simulink model "sbvf_model_2019b_distributed"  (R2019b)
settings: Solver=VariableStepAuto  StartTime=0.0  StopTime=Tsim  RelTol=1e-3
undefined symbols (not defined in the file): A, A0, Ad, B, C, c, D, F, F_dist, Gdiag, k, K, K0, L_leader, std_dev, x0, x0_leader
libraries: dspindex x102, simulink x1
(part 1 of 2)
settings Model: Creator=andre  LastModifiedBy=frare
settings DebuggingCC: UnconnectedInputMsg=none  UnconnectedOutputMsg=none  UnconnectedLineMsg=none
settings ModelReferenceCC: EnableRefExpFcnMdlSchedulingChecks=off
settings RTWCC: Description=Generic Real-Time Target

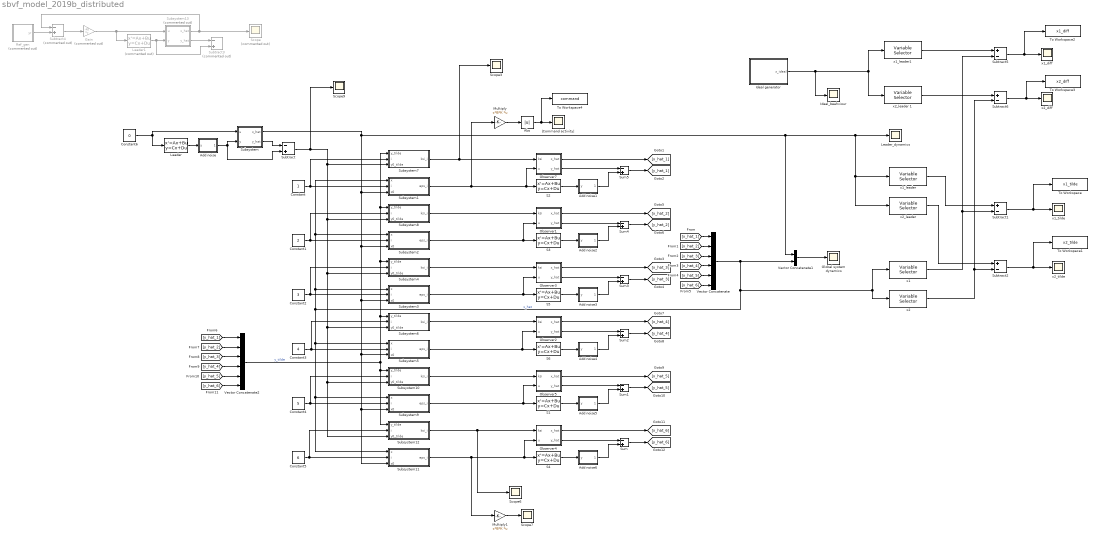
== system sbvf_model_2019b_distributed ==
  Abs : Abs
  Add noise : Subsystem
  "Add noise1 " : Subsystem
  Add noise2 : Subsystem
  Add noise3 : Subsystem
  Add noise4 : Subsystem
  Add noise5 : Subsystem
  Add noise6 : Subsystem
  Constant : Constant
  Constant1 : Constant  Value=2
  Constant2 : Constant  Value=3
  Constant3 : Constant  Value=4
  Constant4 : Constant  Value=5
  Constant5 : Constant  Value=6
  Constant6 : Constant  Value=0
  Gain : Gain  Commented=on  Gain=-K0  Multiplication=Matrix(K*u)
  Global system dynamics : Scope
  "Ideal generator " : Subsystem
  "Ideal_beahviour " : Scope
  Leader : StateSpace  A=A0  B=B  C=C  D=0  InitialCondition=x0_leader
  Leader1 : StateSpace  Commented=on  A=A  B=B  C=C  D=0  InitialCondition=x0_leader
  "Leader_dynamics " : Scope
  Multiply : Gain  Gain=c*B*K  Multiplication=Matrix(K*u)
  Multiply1 : Gain  Gain=c*B*K  Multiplication=Matrix(K*u)
  Observer1 : Subsystem
  Observer2 : Subsystem
  Observer3 : Subsystem
  Observer4 : Subsystem
  Observer5 : Subsystem
  Observer7 : Subsystem
  Ref_gen : Subsystem  Commented=on
  S1 : StateSpace  A=A0  B=c*B*K  C=C  D=D  InitialCondition=x0(:,5)
  S2 : StateSpace  A=A0  B=c*B*K  C=C  D=D  InitialCondition=x0(:,1)
  S3 : StateSpace  A=A0  B=c*B*K  C=C  D=D  InitialCondition=x0(:,2)
  S4 : StateSpace  A=A0  B=c*B*K  C=C  D=D  InitialCondition=x0(:,6)
  S5 : StateSpace  A=A0  B=c*B*K  C=C  D=D  InitialCondition=x0(:,3)
  S6 : StateSpace  A=A0  B=c*B*K  C=C  D=D  InitialCondition=x0(:,4)
  Scope : Scope  Commented=on
  Scope{3,6..7,9} (4 alike) : Scope
  Subsystem : Subsystem
  Subsystem1 : Subsystem
  Subsystem10 : Subsystem
  Subsystem11 : Subsystem
  Subsystem12 : Subsystem
  Subsystem13 : Subsystem  Commented=on
  Subsystem2 : Subsystem
  Subsystem3 : Subsystem
  Subsystem4 : Subsystem
  Subsystem5 : Subsystem
  Subsystem6 : Subsystem
  Subsystem7 : Subsystem
  Subsystem8 : Subsystem
  Subsystem9 : Subsystem
  Subtract : Sum  Inputs=-+
  Subtract{1..2,5..6} (4 alike) : Sum  Inputs=+-
  Subtract3 : Sum  Commented=on  Inputs=-+
  Subtract4 : Sum  Commented=on  Inputs=-+
  Sum{,1..5} (6 alike) : Sum  Inputs=-+
  To Workspace : ToWorkspace  VariableName=x1_tilde  SaveFormat=Timeseries  SampleTime=-1
  To Workspace1 : ToWorkspace  VariableName=x2_tilde  SaveFormat=Timeseries  SampleTime=-1
  To Workspace2 : ToWorkspace  VariableName=x1_diff  SaveFormat=Timeseries  SampleTime=-1
  To Workspace3 : ToWorkspace  VariableName=x2_diff  SaveFormat=Timeseries  SampleTime=-1
  To Workspace4 : ToWorkspace  VariableName=command  SaveFormat=Timeseries  SampleTime=-1
  Vector Concatenate : Concatenate  NumInputs=6  Mode=Multidimensional array  ConcatenateDimension=2
  Vector Concatenate1 : Concatenate  Mode=Multidimensional array  ConcatenateDimension=2
  Vector Concatenate2 : Concatenate  NumInputs=6  Mode=Multidimensional array  ConcatenateDimension=2
  x1 : dspindex/Variable Selector  NumInputs=1  rowsOrCols=Rows  IdxMode=Fixed  Elements=1  ZerOneIdxMode=One-based  errmode=Clip Index  FillMode=on  FillValues=0
  "x1_diff " : Scope
  x1_leader : dspindex/Variable Selector  NumInputs=1  rowsOrCols=Rows  IdxMode=Fixed  Elements=1  ZerOneIdxMode=One-based  errmode=Clip Index  FillMode=on  FillValues=0
  x1_leader1 : dspindex/Variable Selector  NumInputs=1  rowsOrCols=Rows  IdxMode=Fixed  Elements=1  ZerOneIdxMode=One-based  errmode=Clip Index  FillMode=on  FillValues=0
  x1_tilde : Scope
  x2 : dspindex/Variable Selector  NumInputs=1  rowsOrCols=Rows  IdxMode=Fixed  Elements=2  ZerOneIdxMode=One-based  errmode=Clip Index  FillMode=on  FillValues=0
  x2_diff : Scope
  "x2_leader " : dspindex/Variable Selector  NumInputs=1  rowsOrCols=Rows  IdxMode=Fixed  Elements=2  ZerOneIdxMode=One-based  errmode=Clip Index  FillMode=on  FillValues=0
  x2_leader 1 : dspindex/Variable Selector  NumInputs=1  rowsOrCols=Rows  IdxMode=Fixed  Elements=2  ZerOneIdxMode=One-based  errmode=Clip Index  FillMode=on  FillValues=0
  "x2_tilde " : Scope
  "|Command activity| " : Scope
  wires:
  Constant/1 -> Subsystem7/2(i), Subsystem1/2(i)
  Constant1/1 -> Subsystem8/2(i), Subsystem2/2(i)
  Vector Concatenate/1 -> Subsystem1/1(x), Subsystem2/1(x), Subsystem3/1(x), Subsystem11/1(x), Subsystem9/1(x), Subsystem5/1(x), x2/1, x1/1, Vector Concatenate1/2  "x_hat"
  Vector Concatenate1/1 -> Global system dynamics/1
  Constant3/1 -> Subsystem6/2(i), Subsystem5/2(i)
  Constant5/1 -> Subsystem12/2(i), Subsystem11/2(i)
  Constant4/1 -> Subsystem10/2(i), Subsystem9/2(i)
  Constant2/1 -> Subsystem4/2(i), Subsystem3/2(i)
  Subsystem2/1(eps_i) -> S3/1, Observer1/2(u)
  Subsystem3/1(eps_i) -> Observer3/2(u), S5/1
  Subsystem5/1(eps_i) -> S6/1, Observer2/2(u)
  Subsystem9/1(eps_i) -> S1/1, Observer5/2(u)
  Subsystem/2(y_hat) -> Subtract/1
  Subsystem7/1(ksi_i) -> Scope3/1, Observer7/1("ksi ")
  Subsystem10/1(ksi_i) -> Observer5/1("ksi ")
  Subsystem6/1(ksi_i) -> Observer2/1("ksi ")
  Subsystem4/1(ksi_i) -> Observer3/1("ksi ")
  Subsystem8/1(ksi_i) -> Observer1/1("ksi ")
  Observer4/2(y_hat) -> Sum/1
  Observer5/2(y_hat) -> Sum1/1
  Observer2/2(y_hat) -> Sum2/1
  Observer3/2(y_hat) -> Sum3/1
  Observer1/2(y_hat) -> Sum4/1
  Observer7/2(y_hat) -> Sum5/1
  Sum5/1 -> [y_hat_1]
  Observer7/1(x_hat) -> [x_hat_1]
  Observer1/1(x_hat) -> [x_hat_2]
  Sum4/1 -> [y_hat_2]
  Observer3/1(x_hat) -> [x_hat_3]
  Sum3/1 -> [y_hat_3]
  Observer2/1(x_hat) -> [x_hat_4]
  Sum2/1 -> [y_hat_4]
  Observer5/1(x_hat) -> [x_hat_5]
  Sum1/1 -> [y_hat_5]
  Observer4/1(x_hat) -> [x_hat_6]
  Sum/1 -> [y_hat_6]
  [x_hat_1] -> Vector Concatenate/1
  [x_hat_2] -> Vector Concatenate/2
  [x_hat_3] -> Vector Concatenate/3
  [x_hat_4] -> Vector Concatenate/4
  [x_hat_5] -> Vector Concatenate/5
  [x_hat_6] -> Vector Concatenate/6
  [y_hat_2] -> Vector Concatenate2/2
  [y_hat_1] -> Vector Concatenate2/1
  [y_hat_5] -> Vector Concatenate2/5
  [y_hat_3] -> Vector Concatenate2/3
  [y_hat_6] -> Vector Concatenate2/6
  [y_hat_4] -> Vector Concatenate2/4
  Vector Concatenate2/1 -> Subsystem7/1("y_tilde "), Subsystem8/1("y_tilde "), Subsystem4/1("y_tilde "), Subsystem6/1("y_tilde "), Subsystem12/1("y_tilde "), Subsystem10/1("y_tilde ")  "y_tilde"
  Subsystem1/1(eps_i) -> Multiply/1, S2/1, Observer7/2(u)
  Subsystem12/1(ksi_i) -> Observer4/1("ksi "), Scope6/1
  Subsystem11/1(eps_i) -> Multiply1/1, Observer4/2(u), S4/1
  Subtract/1 -> Scope9/1, Subsystem12/3("y0_tilde "), Subsystem10/3("y0_tilde "), Subsystem6/3("y0_tilde "), Subsystem4/3("y0_tilde "), Subsystem8/3("y0_tilde "), Subsystem7/3("y0_tilde ")
  Subsystem/1(x_hat) -> Subsystem11/3(x0), Subsystem9/3(x0), Subsystem5/3(x0), Subsystem3/3(x0), Subsystem2/3(x0), Subsystem1/3(x0), Vector Concatenate1/1, "Leader_dynamics "/1, "x2_leader "/1, x1_leader/1
  x1_leader/1 -> Subtract1/1
  x1/1 -> Subtract5/2, Subtract1/2
  "x2_leader "/1 -> Subtract2/1
  x2/1 -> Subtract6/2, Subtract2/2
  Subtract1/1 -> To Workspace/1, x1_tilde/1
  Constant6/1 -> Subsystem/1(u), Leader/1
  Leader1/1 -> Subtract3/2, Subsystem13/2("y ")
  Subtract4/1 -> Gain/1
  Subsystem13/2(y_hat) -> Subtract3/1
  Subsystem13/1(x_hat) -> Subtract4/1, Scope/1
  Ref_gen/1(yr) -> Subtract4/2
  Gain/1 -> Subsystem13/1(u), Leader1/1
  Subtract2/1 -> To Workspace1/1, "x2_tilde "/1
  "Add noise1 "/1(y_noisy) -> Sum5/2
  Add noise2/1(y_noisy) -> Sum4/2
  Add noise3/1(y_noisy) -> Sum3/2
  Add noise4/1(y_noisy) -> Sum2/2
  Add noise5/1(y_noisy) -> Sum1/2
  Add noise6/1(y_noisy) -> Sum/2
  Add noise/1(y_noisy) -> Subtract/2, Subsystem/2("y ")
  Leader/1 -> Add noise/1(y)
  S3/1 -> Add noise2/1(y)
  S2/1 -> "Add noise1 "/1(y)
  S5/1 -> Add noise3/1(y)
  S6/1 -> Add noise4/1(y)
  S1/1 -> Add noise5/1(y)
  S4/1 -> Add noise6/1(y)
  "Ideal generator "/1("x_ideal ") -> "Ideal_beahviour "/1, x2_leader 1/1, x1_leader1/1
  x1_leader1/1 -> Subtract5/1
  x2_leader 1/1 -> Subtract6/1
  Subtract5/1 -> To Workspace2/1, "x1_diff "/1
  Subtract6/1 -> To Workspace3/1, x2_diff/1
  Multiply/1 -> Abs/1
  Multiply1/1 -> Scope7/1
  Abs/1 -> To Workspace4/1, "|Command activity| "/1

== system sbvf_model_2019b_distributed/Add noise ==
  y : Inport
  Random Number : RandomNumber  SampleTime=0.1
  Sum : Sum  Inputs=|++
  "std_dev(k) " : Gain  Gain=std_dev(k)
  y_noisy : Outport
  wires:
  Random Number/1 -> "std_dev(k) "/1
  y/1 -> Sum/1
  "std_dev(k) "/1 -> Sum/2
  Sum/1 -> y_noisy/1

== system sbvf_model_2019b_distributed/Add noise1  ==
  y : Inport
  Random Number : RandomNumber  SampleTime=0.1
  Sum : Sum  Inputs=|++
  "std_dev(k) " : Gain  Gain=std_dev(k)
  y_noisy : Outport
  wires:
  Random Number/1 -> "std_dev(k) "/1
  y/1 -> Sum/1
  "std_dev(k) "/1 -> Sum/2
  Sum/1 -> y_noisy/1

== system sbvf_model_2019b_distributed/Add noise2 ==
  y : Inport
  Random Number : RandomNumber  SampleTime=0.1
  Sum : Sum  Inputs=|++
  "std_dev(k) " : Gain  Gain=std_dev(k)
  y_noisy : Outport
  wires:
  Random Number/1 -> "std_dev(k) "/1
  y/1 -> Sum/1
  "std_dev(k) "/1 -> Sum/2
  Sum/1 -> y_noisy/1

== system sbvf_model_2019b_distributed/Add noise3 ==
  y : Inport
  Random Number : RandomNumber  SampleTime=0.1
  Sum : Sum  Inputs=|++
  "std_dev(k) " : Gain  Gain=std_dev(k)
  y_noisy : Outport
  wires:
  Random Number/1 -> "std_dev(k) "/1
  y/1 -> Sum/1
  "std_dev(k) "/1 -> Sum/2
  Sum/1 -> y_noisy/1

== system sbvf_model_2019b_distributed/Add noise4 ==
  y : Inport
  Random Number : RandomNumber  SampleTime=0.1
  Sum : Sum  Inputs=|++
  "std_dev(k) " : Gain  Gain=std_dev(k)
  y_noisy : Outport
  wires:
  Random Number/1 -> "std_dev(k) "/1
  y/1 -> Sum/1
  "std_dev(k) "/1 -> Sum/2
  Sum/1 -> y_noisy/1

== system sbvf_model_2019b_distributed/Add noise5 ==
  y : Inport
  Random Number : RandomNumber  SampleTime=0.1
  Sum : Sum  Inputs=|++
  "std_dev(k) " : Gain  Gain=std_dev(k)
  y_noisy : Outport
  wires:
  Random Number/1 -> "std_dev(k) "/1
  y/1 -> Sum/1
  "std_dev(k) "/1 -> Sum/2
  Sum/1 -> y_noisy/1

== system sbvf_model_2019b_distributed/Add noise6 ==
  y : Inport
  Random Number : RandomNumber  SampleTime=0.1
  Sum : Sum  Inputs=|++
  "std_dev(k) " : Gain  Gain=std_dev(k)
  y_noisy : Outport
  wires:
  Random Number/1 -> "std_dev(k) "/1
  y/1 -> Sum/1
  "std_dev(k) "/1 -> Sum/2
  Sum/1 -> y_noisy/1

== system sbvf_model_2019b_distributed/Ideal generator  ==
  Constant7 : Constant  Value=0
  Leader2 : StateSpace  A=A0  B=B  C=C  D=0  InitialCondition=x0_leader
  Subsystem14 : Subsystem
  "x_ideal " : Outport
  wires:
  Constant7/1 -> Subsystem14/1(u), Leader2/1
  Leader2/1 -> Subsystem14/2("y ")
  Subsystem14/1(x_hat) -> "x_ideal "/1

== system sbvf_model_2019b_distributed/Observer1 ==
  "ksi " : Inport
  u : Inport  Port=2
  Add1 : Sum  Inputs=+++
  Gain : Gain  Gain=-c*F_dist  Multiplication=Matrix(K*u)
  Gain1 : Gain  Gain=c*B*K  Multiplication=Matrix(K*u)
  Gain2 : Gain  Gain=A0  Multiplication=Matrix(K*u)
  Gain3 : Gain  Gain=C  Multiplication=Matrix(K*u)
  Integrator : Integrator  InitialCondition=x0(:,2)
  x_hat : Outport
  y_hat : Outport  Port=2
  wires:
  Gain2/1 -> Add1/3
  Gain/1 -> Add1/2
  Integrator/1 -> x_hat/1, Gain2/1, Gain3/1  "x_hat"
  Add1/1 -> Integrator/1
  u/1 -> Gain1/1
  Gain1/1 -> Add1/1
  "ksi "/1 -> Gain/1
  Gain3/1 -> y_hat/1

== system sbvf_model_2019b_distributed/Observer2 ==
  "ksi " : Inport
  u : Inport  Port=2
  Add1 : Sum  Inputs=+++
  Gain : Gain  Gain=-c*F_dist  Multiplication=Matrix(K*u)
  Gain1 : Gain  Gain=c*B*K  Multiplication=Matrix(K*u)
  Gain2 : Gain  Gain=A0  Multiplication=Matrix(K*u)
  Gain3 : Gain  Gain=C  Multiplication=Matrix(K*u)
  Integrator : Integrator  InitialCondition=x0(:,4)
  x_hat : Outport
  y_hat : Outport  Port=2
  wires:
  Gain2/1 -> Add1/3
  Gain/1 -> Add1/2
  Integrator/1 -> x_hat/1, Gain2/1, Gain3/1  "x_hat"
  Add1/1 -> Integrator/1
  u/1 -> Gain1/1
  Gain1/1 -> Add1/1
  "ksi "/1 -> Gain/1
  Gain3/1 -> y_hat/1

== system sbvf_model_2019b_distributed/Observer3 ==
  "ksi " : Inport
  u : Inport  Port=2
  Add1 : Sum  Inputs=+++
  Gain : Gain  Gain=-c*F_dist  Multiplication=Matrix(K*u)
  Gain1 : Gain  Gain=c*B*K  Multiplication=Matrix(K*u)
  Gain2 : Gain  Gain=A0  Multiplication=Matrix(K*u)
  Gain3 : Gain  Gain=C  Multiplication=Matrix(K*u)
  Integrator : Integrator  InitialCondition=x0(:,3)
  x_hat : Outport
  y_hat : Outport  Port=2
  wires:
  Gain2/1 -> Add1/3
  Gain/1 -> Add1/2
  Integrator/1 -> x_hat/1, Gain2/1, Gain3/1  "x_hat"
  Add1/1 -> Integrator/1
  u/1 -> Gain1/1
  Gain1/1 -> Add1/1
  "ksi "/1 -> Gain/1
  Gain3/1 -> y_hat/1

== system sbvf_model_2019b_distributed/Observer4 ==
  "ksi " : Inport
  u : Inport  Port=2
  Add1 : Sum  Inputs=+++
  Gain : Gain  Gain=-c*F_dist  Multiplication=Matrix(K*u)
  Gain1 : Gain  Gain=c*B*K  Multiplication=Matrix(K*u)
  Gain2 : Gain  Gain=A0  Multiplication=Matrix(K*u)
  Gain3 : Gain  Gain=C  Multiplication=Matrix(K*u)
  Integrator : Integrator  InitialCondition=x0(:,6)
  x_hat : Outport
  y_hat : Outport  Port=2
  wires:
  Gain2/1 -> Add1/3
  Gain/1 -> Add1/2
  Integrator/1 -> x_hat/1, Gain2/1, Gain3/1  "x_hat"
  Add1/1 -> Integrator/1
  u/1 -> Gain1/1
  Gain1/1 -> Add1/1
  "ksi "/1 -> Gain/1
  Gain3/1 -> y_hat/1

== system sbvf_model_2019b_distributed/Observer5 ==
  "ksi " : Inport
  u : Inport  Port=2
  Add1 : Sum  Inputs=+++
  Gain : Gain  Gain=-c*F_dist  Multiplication=Matrix(K*u)
  Gain1 : Gain  Gain=c*B*K  Multiplication=Matrix(K*u)
  Gain2 : Gain  Gain=A0  Multiplication=Matrix(K*u)
  Gain3 : Gain  Gain=C  Multiplication=Matrix(K*u)
  Integrator : Integrator  InitialCondition=x0(:,5)
  x_hat : Outport
  y_hat : Outport  Port=2
  wires:
  Gain2/1 -> Add1/3
  Gain/1 -> Add1/2
  Integrator/1 -> x_hat/1, Gain2/1, Gain3/1  "x_hat"
  Add1/1 -> Integrator/1
  u/1 -> Gain1/1
  Gain1/1 -> Add1/1
  "ksi "/1 -> Gain/1
  Gain3/1 -> y_hat/1

== system sbvf_model_2019b_distributed/Observer7 ==
  "ksi " : Inport
  u : Inport  Port=2
  Add1 : Sum  Inputs=+++
  Gain : Gain  Gain=-c*F_dist  Multiplication=Matrix(K*u)
  Gain1 : Gain  Gain=c*B*K  Multiplication=Matrix(K*u)
  Gain2 : Gain  Gain=A0  Multiplication=Matrix(K*u)
  Gain3 : Gain  Gain=C  Multiplication=Matrix(K*u)
  Integrator : Integrator  InitialCondition=x0(:,1)
  x_hat : Outport
  y_hat : Outport  Port=2
  wires:
  Gain2/1 -> Add1/3
  Gain/1 -> Add1/2
  Integrator/1 -> x_hat/1, Gain2/1, Gain3/1  "x_hat"
  Add1/1 -> Integrator/1
  u/1 -> Gain1/1
  Gain1/1 -> Add1/1
  "ksi "/1 -> Gain/1
  Gain3/1 -> y_hat/1

== system sbvf_model_2019b_distributed/Ref_gen ==
  Derivative : Derivative
  Mux : Mux  Inputs=2
  Ramp : simulink/Sources/Ramp  slope=1  start=0  InitialOutput=0
  yr : Outport
  wires:
  Mux/1 -> yr/1
  Ramp/1 -> Derivative/1, Mux/1
  Derivative/1 -> Mux/2

== system sbvf_model_2019b_distributed/Subsystem ==
  u : Inport
  "y " : Inport  Port=2
  Add1 : Sum  Inputs=+++
  Gain : Gain  Gain=c*L_leader  Multiplication=Matrix(K*u)
  Gain1 : Gain  Gain=B  Multiplication=Matrix(K*u)
  Gain2 : Gain  Gain=A0  Multiplication=Matrix(K*u)
  Gain3 : Gain  Gain=C  Multiplication=Matrix(K*u)
  Integrator : Integrator  InitialCondition=x0_leader
  Subtract : Sum  Inputs=-+
  x_hat : Outport
  y_hat : Outport  Port=2
  wires:
  Gain2/1 -> Add1/3
  Gain/1 -> Add1/2
  Integrator/1 -> x_hat/1, Gain3/1, Gain2/1  "x_hat"
  Add1/1 -> Integrator/1  "x_hat_dot"
  u/1 -> Gain1/1
  Gain1/1 -> Add1/1
  "y "/1 -> Subtract/2
  Subtract/1 -> Gain/1
  Gain3/1 -> y_hat/1, Subtract/1

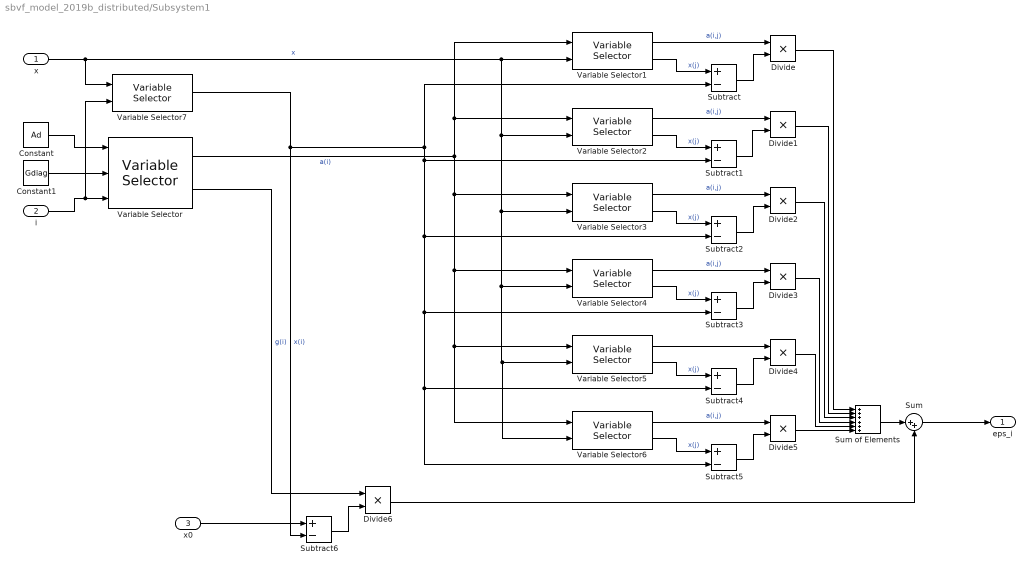
== system sbvf_model_2019b_distributed/Subsystem1 ==
  x : Inport
  i : Inport  Port=2
  x0 : Inport  Port=3
  Constant : Constant  Value=Ad
  Constant1 : Constant  Value=Gdiag
  Divide{,1..6} (7 alike) : Product
  Subtract{,1..6} (7 alike) : Sum  Inputs=+-
  Sum : Sum  Inputs=|++
  Sum of Elements : Sum  Inputs=++++++
  Variable Selector : dspindex/Variable Selector  NumInputs=2  rowsOrCols=Rows  IdxMode=Variable  Elements=[1 3]  ZerOneIdxMode=One-based  errmode=Clip and Warn  FillMode=on  FillValues=0
  Variable Selector1 : dspindex/Variable Selector  NumInputs=2  rowsOrCols=Columns  IdxMode=Fixed  Elements=1  ZerOneIdxMode=One-based  errmode=Generate Error  FillMode=on  FillValues=0
  Variable Selector2 : dspindex/Variable Selector  NumInputs=2  rowsOrCols=Columns  IdxMode=Fixed  Elements=2  ZerOneIdxMode=One-based  errmode=Generate Error  FillMode=on  FillValues=0
  Variable Selector3 : dspindex/Variable Selector  NumInputs=2  rowsOrCols=Columns  IdxMode=Fixed  Elements=3  ZerOneIdxMode=One-based  errmode=Generate Error  FillMode=on  FillValues=0
  Variable Selector4 : dspindex/Variable Selector  NumInputs=2  rowsOrCols=Columns  IdxMode=Fixed  Elements=4  ZerOneIdxMode=One-based  errmode=Generate Error  FillMode=on  FillValues=0
  Variable Selector5 : dspindex/Variable Selector  NumInputs=2  rowsOrCols=Columns  IdxMode=Fixed  Elements=5  ZerOneIdxMode=One-based  errmode=Generate Error  FillMode=on  FillValues=0
  Variable Selector6 : dspindex/Variable Selector  NumInputs=2  rowsOrCols=Columns  IdxMode=Fixed  Elements=6  ZerOneIdxMode=One-based  errmode=Generate Error  FillMode=on  FillValues=0
  Variable Selector7 : dspindex/Variable Selector  NumInputs=1  rowsOrCols=Columns  IdxMode=Variable  Elements=1  ZerOneIdxMode=One-based  errmode=Generate Error  FillMode=on  FillValues=0
  eps_i : Outport
  wires:
  Variable Selector/1 -> Variable Selector3/1, Variable Selector4/1, Variable Selector6/1, Variable Selector5/1, Variable Selector2/1, Variable Selector1/1  "a(i)"
  x/1 -> Variable Selector7/1, Variable Selector2/2, Variable Selector3/2, Variable Selector4/2, Variable Selector6/2, Variable Selector5/2, Variable Selector1/2  "x"
  Constant/1 -> Variable Selector/1
  i/1 -> Variable Selector7/2, Variable Selector/3
  Variable Selector1/1 -> Divide/1  "a(i,j)"
  Variable Selector1/2 -> Subtract/1  "x(j)"
  Subtract/1 -> Divide/2
  Variable Selector2/2 -> Subtract1/1  "x(j)"
  Variable Selector2/1 -> Divide1/1  "a(i,j)"
  Subtract1/1 -> Divide1/2
  Variable Selector3/1 -> Divide2/1  "a(i,j)"
  Variable Selector3/2 -> Subtract2/1  "x(j)"
  Subtract2/1 -> Divide2/2
  Variable Selector4/1 -> Divide3/1  "a(i,j)"
  Variable Selector4/2 -> Subtract3/1  "x(j)"
  Subtract3/1 -> Divide3/2
  Variable Selector5/2 -> Subtract4/1  "x(j)"
  Subtract4/1 -> Divide4/2
  Variable Selector5/1 -> Divide4/1
  Variable Selector6/1 -> Divide5/1  "a(i,j)"
  Variable Selector7/1 -> Subtract6/2, Subtract5/2, Subtract4/2, Subtract3/2, Subtract2/2, Subtract1/2, Subtract/2  "x(i)"
  Variable Selector6/2 -> Subtract5/1  "x(j)"
  Subtract5/1 -> Divide5/2
  Divide2/1 -> Sum of Elements/3
  Divide1/1 -> Sum of Elements/2
  Divide5/1 -> Sum of Elements/6
  Divide4/1 -> Sum of Elements/5
  Divide3/1 -> Sum of Elements/4
  Divide/1 -> Sum of Elements/1
  Variable Selector/2 -> Divide6/1  "g(i)"
  Subtract6/1 -> Divide6/2
  x0/1 -> Subtract6/1
  Divide6/1 -> Sum/2
  Sum of Elements/1 -> Sum/1
  Sum/1 -> eps_i/1
  Constant1/1 -> Variable Selector/2

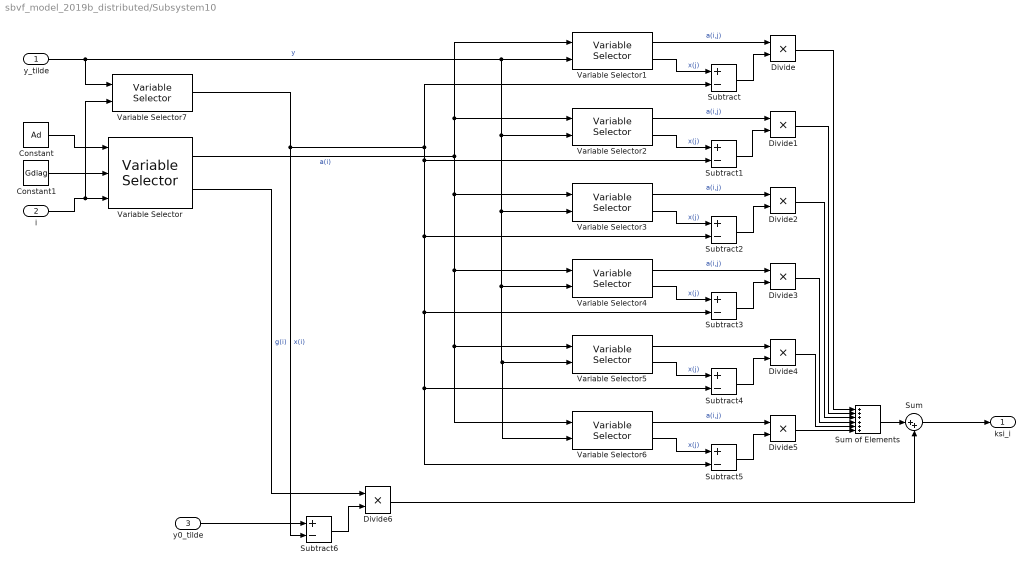
== system sbvf_model_2019b_distributed/Subsystem10 ==
  "y_tilde " : Inport
  i : Inport  Port=2
  "y0_tilde " : Inport  Port=3
  Constant : Constant  Value=Ad
  Constant1 : Constant  Value=Gdiag
  Divide{,1..6} (7 alike) : Product
  Subtract{,1..6} (7 alike) : Sum  Inputs=+-
  Sum : Sum  Inputs=|++
  Sum of Elements : Sum  Inputs=++++++
  Variable Selector : dspindex/Variable Selector  NumInputs=2  rowsOrCols=Rows  IdxMode=Variable  Elements=[1 3]  ZerOneIdxMode=One-based  errmode=Clip and Warn  FillMode=on  FillValues=0
  Variable Selector1 : dspindex/Variable Selector  NumInputs=2  rowsOrCols=Columns  IdxMode=Fixed  Elements=1  ZerOneIdxMode=One-based  errmode=Generate Error  FillMode=on  FillValues=0
  Variable Selector2 : dspindex/Variable Selector  NumInputs=2  rowsOrCols=Columns  IdxMode=Fixed  Elements=2  ZerOneIdxMode=One-based  errmode=Generate Error  FillMode=on  FillValues=0
  Variable Selector3 : dspindex/Variable Selector  NumInputs=2  rowsOrCols=Columns  IdxMode=Fixed  Elements=3  ZerOneIdxMode=One-based  errmode=Generate Error  FillMode=on  FillValues=0
  Variable Selector4 : dspindex/Variable Selector  NumInputs=2  rowsOrCols=Columns  IdxMode=Fixed  Elements=4  ZerOneIdxMode=One-based  errmode=Generate Error  FillMode=on  FillValues=0
  Variable Selector5 : dspindex/Variable Selector  NumInputs=2  rowsOrCols=Columns  IdxMode=Fixed  Elements=5  ZerOneIdxMode=One-based  errmode=Generate Error  FillMode=on  FillValues=0
  Variable Selector6 : dspindex/Variable Selector  NumInputs=2  rowsOrCols=Columns  IdxMode=Fixed  Elements=6  ZerOneIdxMode=One-based  errmode=Generate Error  FillMode=on  FillValues=0
  Variable Selector7 : dspindex/Variable Selector  NumInputs=1  rowsOrCols=Columns  IdxMode=Variable  Elements=1  ZerOneIdxMode=One-based  errmode=Generate Error  FillMode=on  FillValues=0
  ksi_i : Outport
  wires:
  Variable Selector/1 -> Variable Selector3/1, Variable Selector4/1, Variable Selector6/1, Variable Selector5/1, Variable Selector2/1, Variable Selector1/1  "a(i)"
  "y_tilde "/1 -> Variable Selector7/1, Variable Selector2/2, Variable Selector3/2, Variable Selector4/2, Variable Selector6/2, Variable Selector5/2, Variable Selector1/2  "y"
  Constant/1 -> Variable Selector/1
  i/1 -> Variable Selector7/2, Variable Selector/3
  Variable Selector1/1 -> Divide/1  "a(i,j)"
  Variable Selector1/2 -> Subtract/1  "x(j)"
  Subtract/1 -> Divide/2
  Variable Selector2/2 -> Subtract1/1  "x(j)"
  Variable Selector2/1 -> Divide1/1  "a(i,j)"
  Subtract1/1 -> Divide1/2
  Variable Selector3/1 -> Divide2/1  "a(i,j)"
  Variable Selector3/2 -> Subtract2/1  "x(j)"
  Subtract2/1 -> Divide2/2
  Variable Selector4/1 -> Divide3/1  "a(i,j)"
  Variable Selector4/2 -> Subtract3/1  "x(j)"
  Subtract3/1 -> Divide3/2
  Variable Selector5/2 -> Subtract4/1  "x(j)"
  Subtract4/1 -> Divide4/2
  Variable Selector5/1 -> Divide4/1
  Variable Selector6/1 -> Divide5/1  "a(i,j)"
  Variable Selector7/1 -> Subtract6/2, Subtract5/2, Subtract4/2, Subtract3/2, Subtract2/2, Subtract1/2, Subtract/2  "x(i)"
  Variable Selector6/2 -> Subtract5/1  "x(j)"
  Subtract5/1 -> Divide5/2
  Divide2/1 -> Sum of Elements/3
  Divide1/1 -> Sum of Elements/2
  Divide5/1 -> Sum of Elements/6
  Divide4/1 -> Sum of Elements/5
  Divide3/1 -> Sum of Elements/4
  Divide/1 -> Sum of Elements/1
  Variable Selector/2 -> Divide6/1  "g(i)"
  Subtract6/1 -> Divide6/2
  "y0_tilde "/1 -> Subtract6/1
  Divide6/1 -> Sum/2
  Sum of Elements/1 -> Sum/1
  Sum/1 -> ksi_i/1
  Constant1/1 -> Variable Selector/2

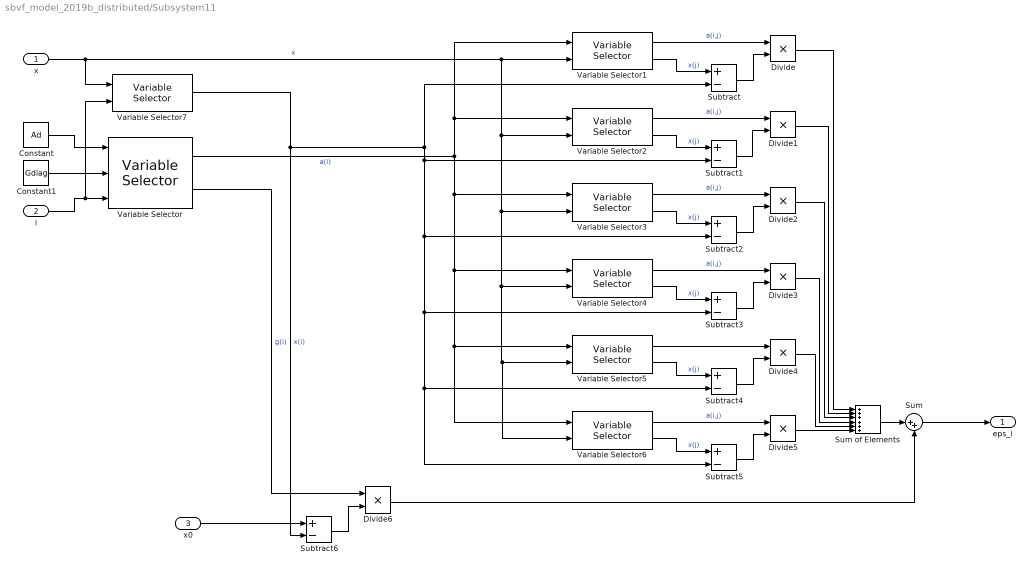
== system sbvf_model_2019b_distributed/Subsystem11 ==
  x : Inport
  i : Inport  Port=2
  x0 : Inport  Port=3
  Constant : Constant  Value=Ad
  Constant1 : Constant  Value=Gdiag
  Divide{,1..6} (7 alike) : Product
  Subtract{,1..6} (7 alike) : Sum  Inputs=+-
  Sum : Sum  Inputs=|++
  Sum of Elements : Sum  Inputs=++++++
  Variable Selector : dspindex/Variable Selector  NumInputs=2  rowsOrCols=Rows  IdxMode=Variable  Elements=[1 3]  ZerOneIdxMode=One-based  errmode=Clip and Warn  FillMode=on  FillValues=0
  Variable Selector1 : dspindex/Variable Selector  NumInputs=2  rowsOrCols=Columns  IdxMode=Fixed  Elements=1  ZerOneIdxMode=One-based  errmode=Generate Error  FillMode=on  FillValues=0
  Variable Selector2 : dspindex/Variable Selector  NumInputs=2  rowsOrCols=Columns  IdxMode=Fixed  Elements=2  ZerOneIdxMode=One-based  errmode=Generate Error  FillMode=on  FillValues=0
  Variable Selector3 : dspindex/Variable Selector  NumInputs=2  rowsOrCols=Columns  IdxMode=Fixed  Elements=3  ZerOneIdxMode=One-based  errmode=Generate Error  FillMode=on  FillValues=0
  Variable Selector4 : dspindex/Variable Selector  NumInputs=2  rowsOrCols=Columns  IdxMode=Fixed  Elements=4  ZerOneIdxMode=One-based  errmode=Generate Error  FillMode=on  FillValues=0
  Variable Selector5 : dspindex/Variable Selector  NumInputs=2  rowsOrCols=Columns  IdxMode=Fixed  Elements=5  ZerOneIdxMode=One-based  errmode=Generate Error  FillMode=on  FillValues=0
  Variable Selector6 : dspindex/Variable Selector  NumInputs=2  rowsOrCols=Columns  IdxMode=Fixed  Elements=6  ZerOneIdxMode=One-based  errmode=Generate Error  FillMode=on  FillValues=0
  Variable Selector7 : dspindex/Variable Selector  NumInputs=1  rowsOrCols=Columns  IdxMode=Variable  Elements=1  ZerOneIdxMode=One-based  errmode=Generate Error  FillMode=on  FillValues=0
  eps_i : Outport
  wires:
  Variable Selector/1 -> Variable Selector3/1, Variable Selector4/1, Variable Selector6/1, Variable Selector5/1, Variable Selector2/1, Variable Selector1/1  "a(i)"
  x/1 -> Variable Selector7/1, Variable Selector2/2, Variable Selector3/2, Variable Selector4/2, Variable Selector6/2, Variable Selector5/2, Variable Selector1/2  "x"
  Constant/1 -> Variable Selector/1
  i/1 -> Variable Selector7/2, Variable Selector/3
  Variable Selector1/1 -> Divide/1  "a(i,j)"
  Variable Selector1/2 -> Subtract/1  "x(j)"
  Subtract/1 -> Divide/2
  Variable Selector2/2 -> Subtract1/1  "x(j)"
  Variable Selector2/1 -> Divide1/1  "a(i,j)"
  Subtract1/1 -> Divide1/2
  Variable Selector3/1 -> Divide2/1  "a(i,j)"
  Variable Selector3/2 -> Subtract2/1  "x(j)"
  Subtract2/1 -> Divide2/2
  Variable Selector4/1 -> Divide3/1  "a(i,j)"
  Variable Selector4/2 -> Subtract3/1  "x(j)"
  Subtract3/1 -> Divide3/2
  Variable Selector5/2 -> Subtract4/1  "x(j)"
  Subtract4/1 -> Divide4/2
  Variable Selector5/1 -> Divide4/1
  Variable Selector6/1 -> Divide5/1  "a(i,j)"
  Variable Selector7/1 -> Subtract6/2, Subtract5/2, Subtract4/2, Subtract3/2, Subtract2/2, Subtract1/2, Subtract/2  "x(i)"
  Variable Selector6/2 -> Subtract5/1  "x(j)"
  Subtract5/1 -> Divide5/2
  Divide2/1 -> Sum of Elements/3
  Divide1/1 -> Sum of Elements/2
  Divide5/1 -> Sum of Elements/6
  Divide4/1 -> Sum of Elements/5
  Divide3/1 -> Sum of Elements/4
  Divide/1 -> Sum of Elements/1
  Variable Selector/2 -> Divide6/1  "g(i)"
  Subtract6/1 -> Divide6/2
  x0/1 -> Subtract6/1
  Divide6/1 -> Sum/2
  Sum of Elements/1 -> Sum/1
  Sum/1 -> eps_i/1
  Constant1/1 -> Variable Selector/2

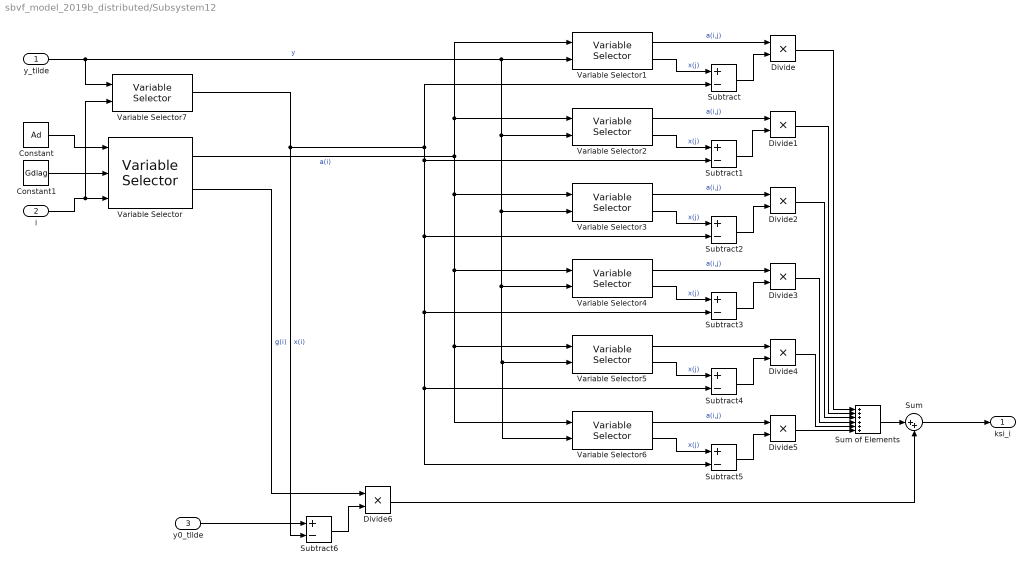
== system sbvf_model_2019b_distributed/Subsystem12 ==
  "y_tilde " : Inport
  i : Inport  Port=2
  "y0_tilde " : Inport  Port=3
  Constant : Constant  Value=Ad
  Constant1 : Constant  Value=Gdiag
  Divide{,1..6} (7 alike) : Product
  Subtract{,1..6} (7 alike) : Sum  Inputs=+-
  Sum : Sum  Inputs=|++
  Sum of Elements : Sum  Inputs=++++++
  Variable Selector : dspindex/Variable Selector  NumInputs=2  rowsOrCols=Rows  IdxMode=Variable  Elements=[1 3]  ZerOneIdxMode=One-based  errmode=Clip and Warn  FillMode=on  FillValues=0
  Variable Selector1 : dspindex/Variable Selector  NumInputs=2  rowsOrCols=Columns  IdxMode=Fixed  Elements=1  ZerOneIdxMode=One-based  errmode=Generate Error  FillMode=on  FillValues=0
  Variable Selector2 : dspindex/Variable Selector  NumInputs=2  rowsOrCols=Columns  IdxMode=Fixed  Elements=2  ZerOneIdxMode=One-based  errmode=Generate Error  FillMode=on  FillValues=0
  Variable Selector3 : dspindex/Variable Selector  NumInputs=2  rowsOrCols=Columns  IdxMode=Fixed  Elements=3  ZerOneIdxMode=One-based  errmode=Generate Error  FillMode=on  FillValues=0
  Variable Selector4 : dspindex/Variable Selector  NumInputs=2  rowsOrCols=Columns  IdxMode=Fixed  Elements=4  ZerOneIdxMode=One-based  errmode=Generate Error  FillMode=on  FillValues=0
  Variable Selector5 : dspindex/Variable Selector  NumInputs=2  rowsOrCols=Columns  IdxMode=Fixed  Elements=5  ZerOneIdxMode=One-based  errmode=Generate Error  FillMode=on  FillValues=0
  Variable Selector6 : dspindex/Variable Selector  NumInputs=2  rowsOrCols=Columns  IdxMode=Fixed  Elements=6  ZerOneIdxMode=One-based  errmode=Generate Error  FillMode=on  FillValues=0
  Variable Selector7 : dspindex/Variable Selector  NumInputs=1  rowsOrCols=Columns  IdxMode=Variable  Elements=1  ZerOneIdxMode=One-based  errmode=Generate Error  FillMode=on  FillValues=0
  ksi_i : Outport
  wires:
  Variable Selector/1 -> Variable Selector3/1, Variable Selector4/1, Variable Selector6/1, Variable Selector5/1, Variable Selector2/1, Variable Selector1/1  "a(i)"
  "y_tilde "/1 -> Variable Selector7/1, Variable Selector2/2, Variable Selector3/2, Variable Selector4/2, Variable Selector6/2, Variable Selector5/2, Variable Selector1/2  "y"
  Constant/1 -> Variable Selector/1
  i/1 -> Variable Selector7/2, Variable Selector/3
  Variable Selector1/1 -> Divide/1  "a(i,j)"
  Variable Selector1/2 -> Subtract/1  "x(j)"
  Subtract/1 -> Divide/2
  Variable Selector2/2 -> Subtract1/1  "x(j)"
  Variable Selector2/1 -> Divide1/1  "a(i,j)"
  Subtract1/1 -> Divide1/2
  Variable Selector3/1 -> Divide2/1  "a(i,j)"
  Variable Selector3/2 -> Subtract2/1  "x(j)"
  Subtract2/1 -> Divide2/2
  Variable Selector4/1 -> Divide3/1  "a(i,j)"
  Variable Selector4/2 -> Subtract3/1  "x(j)"
  Subtract3/1 -> Divide3/2
  Variable Selector5/2 -> Subtract4/1  "x(j)"
  Subtract4/1 -> Divide4/2
  Variable Selector5/1 -> Divide4/1
  Variable Selector6/1 -> Divide5/1  "a(i,j)"
  Variable Selector7/1 -> Subtract6/2, Subtract5/2, Subtract4/2, Subtract3/2, Subtract2/2, Subtract1/2, Subtract/2  "x(i)"
  Variable Selector6/2 -> Subtract5/1  "x(j)"
  Subtract5/1 -> Divide5/2
  Divide2/1 -> Sum of Elements/3
  Divide1/1 -> Sum of Elements/2
  Divide5/1 -> Sum of Elements/6
  Divide4/1 -> Sum of Elements/5
  Divide3/1 -> Sum of Elements/4
  Divide/1 -> Sum of Elements/1
  Variable Selector/2 -> Divide6/1  "g(i)"
  Subtract6/1 -> Divide6/2
  "y0_tilde "/1 -> Subtract6/1
  Divide6/1 -> Sum/2
  Sum of Elements/1 -> Sum/1
  Sum/1 -> ksi_i/1
  Constant1/1 -> Variable Selector/2

== system sbvf_model_2019b_distributed/Subsystem13 ==
  u : Inport
  "y " : Inport  Port=2
  Add1 : Sum  Inputs=+++
  Gain : Gain  Gain=-c*F  Multiplication=Matrix(K*u)
  Gain1 : Gain  Gain=B  Multiplication=Matrix(K*u)
  Gain2 : Gain  Gain=A  Multiplication=Matrix(K*u)
  Gain3 : Gain  Gain=C  Multiplication=Matrix(K*u)
  Integrator : Integrator  InitialCondition=x0_leader
  Subtract : Sum  Inputs=-+
  x_hat : Outport
  y_hat : Outport  Port=2
  wires:
  Gain2/1 -> Add1/3
  Gain/1 -> Add1/2
  Integrator/1 -> x_hat/1, Gain3/1, Gain2/1  "x_hat"
  Add1/1 -> Integrator/1  "x_hat_dot"
  u/1 -> Gain1/1
  Gain1/1 -> Add1/1
  "y "/1 -> Subtract/2
  Subtract/1 -> Gain/1
  Gain3/1 -> y_hat/1, Subtract/1

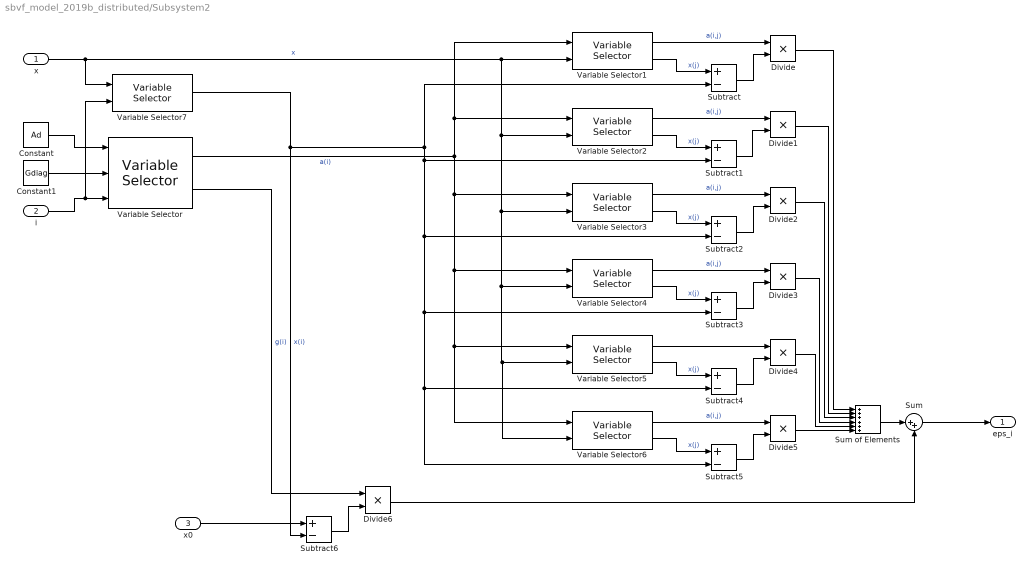
== system sbvf_model_2019b_distributed/Subsystem2 ==
  x : Inport
  i : Inport  Port=2
  x0 : Inport  Port=3
  Constant : Constant  Value=Ad
  Constant1 : Constant  Value=Gdiag
  Divide{,1..6} (7 alike) : Product
  Subtract{,1..6} (7 alike) : Sum  Inputs=+-
  Sum : Sum  Inputs=|++
  Sum of Elements : Sum  Inputs=++++++
  Variable Selector : dspindex/Variable Selector  NumInputs=2  rowsOrCols=Rows  IdxMode=Variable  Elements=[1 3]  ZerOneIdxMode=One-based  errmode=Clip and Warn  FillMode=on  FillValues=0
  Variable Selector1 : dspindex/Variable Selector  NumInputs=2  rowsOrCols=Columns  IdxMode=Fixed  Elements=1  ZerOneIdxMode=One-based  errmode=Generate Error  FillMode=on  FillValues=0
  Variable Selector2 : dspindex/Variable Selector  NumInputs=2  rowsOrCols=Columns  IdxMode=Fixed  Elements=2  ZerOneIdxMode=One-based  errmode=Generate Error  FillMode=on  FillValues=0
  Variable Selector3 : dspindex/Variable Selector  NumInputs=2  rowsOrCols=Columns  IdxMode=Fixed  Elements=3  ZerOneIdxMode=One-based  errmode=Generate Error  FillMode=on  FillValues=0
  Variable Selector4 : dspindex/Variable Selector  NumInputs=2  rowsOrCols=Columns  IdxMode=Fixed  Elements=4  ZerOneIdxMode=One-based  errmode=Generate Error  FillMode=on  FillValues=0
  Variable Selector5 : dspindex/Variable Selector  NumInputs=2  rowsOrCols=Columns  IdxMode=Fixed  Elements=5  ZerOneIdxMode=One-based  errmode=Generate Error  FillMode=on  FillValues=0
  Variable Selector6 : dspindex/Variable Selector  NumInputs=2  rowsOrCols=Columns  IdxMode=Fixed  Elements=6  ZerOneIdxMode=One-based  errmode=Generate Error  FillMode=on  FillValues=0
  Variable Selector7 : dspindex/Variable Selector  NumInputs=1  rowsOrCols=Columns  IdxMode=Variable  Elements=1  ZerOneIdxMode=One-based  errmode=Generate Error  FillMode=on  FillValues=0
  eps_i : Outport
  wires:
  Variable Selector/1 -> Variable Selector3/1, Variable Selector4/1, Variable Selector6/1, Variable Selector5/1, Variable Selector2/1, Variable Selector1/1  "a(i)"
  x/1 -> Variable Selector7/1, Variable Selector2/2, Variable Selector3/2, Variable Selector4/2, Variable Selector6/2, Variable Selector5/2, Variable Selector1/2  "x"
  Constant/1 -> Variable Selector/1
  i/1 -> Variable Selector7/2, Variable Selector/3
  Variable Selector1/1 -> Divide/1  "a(i,j)"
  Variable Selector1/2 -> Subtract/1  "x(j)"
  Subtract/1 -> Divide/2
  Variable Selector2/2 -> Subtract1/1  "x(j)"
  Variable Selector2/1 -> Divide1/1  "a(i,j)"
  Subtract1/1 -> Divide1/2
  Variable Selector3/1 -> Divide2/1  "a(i,j)"
  Variable Selector3/2 -> Subtract2/1  "x(j)"
  Subtract2/1 -> Divide2/2
  Variable Selector4/1 -> Divide3/1  "a(i,j)"
  Variable Selector4/2 -> Subtract3/1  "x(j)"
  Subtract3/1 -> Divide3/2
  Variable Selector5/2 -> Subtract4/1  "x(j)"
  Subtract4/1 -> Divide4/2
  Variable Selector5/1 -> Divide4/1
  Variable Selector6/1 -> Divide5/1  "a(i,j)"
  Variable Selector7/1 -> Subtract6/2, Subtract5/2, Subtract4/2, Subtract3/2, Subtract2/2, Subtract1/2, Subtract/2  "x(i)"
  Variable Selector6/2 -> Subtract5/1  "x(j)"
  Subtract5/1 -> Divide5/2
  Divide2/1 -> Sum of Elements/3
  Divide1/1 -> Sum of Elements/2
  Divide5/1 -> Sum of Elements/6
  Divide4/1 -> Sum of Elements/5
  Divide3/1 -> Sum of Elements/4
  Divide/1 -> Sum of Elements/1
  Variable Selector/2 -> Divide6/1  "g(i)"
  Subtract6/1 -> Divide6/2
  x0/1 -> Subtract6/1
  Divide6/1 -> Sum/2
  Sum of Elements/1 -> Sum/1
  Sum/1 -> eps_i/1
  Constant1/1 -> Variable Selector/2

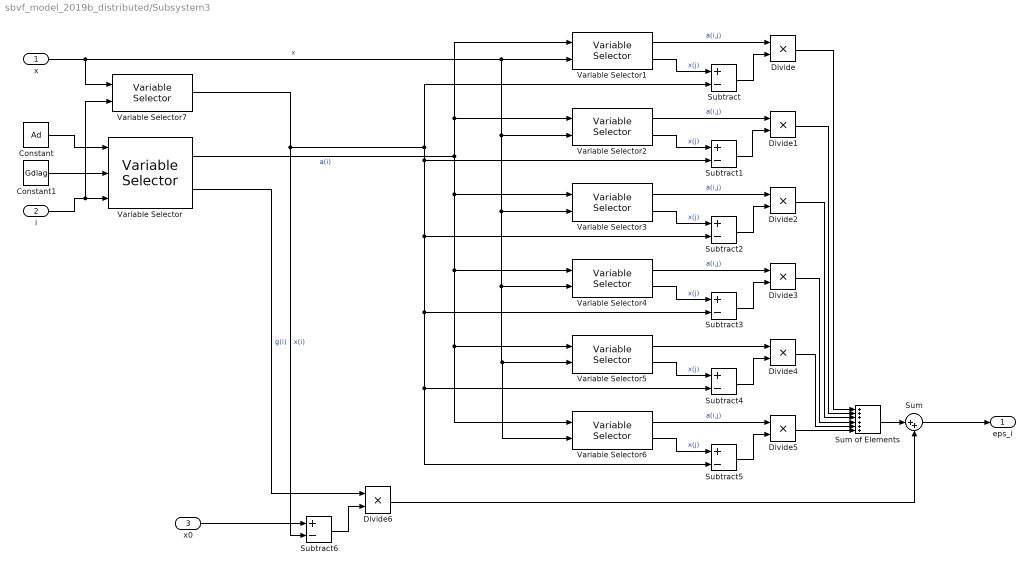
== system sbvf_model_2019b_distributed/Subsystem3 ==
  x : Inport
  i : Inport  Port=2
  x0 : Inport  Port=3
  Constant : Constant  Value=Ad
  Constant1 : Constant  Value=Gdiag
  Divide{,1..6} (7 alike) : Product
  Subtract{,1..6} (7 alike) : Sum  Inputs=+-
  Sum : Sum  Inputs=|++
  Sum of Elements : Sum  Inputs=++++++
  Variable Selector : dspindex/Variable Selector  NumInputs=2  rowsOrCols=Rows  IdxMode=Variable  Elements=[1 3]  ZerOneIdxMode=One-based  errmode=Clip and Warn  FillMode=on  FillValues=0
  Variable Selector1 : dspindex/Variable Selector  NumInputs=2  rowsOrCols=Columns  IdxMode=Fixed  Elements=1  ZerOneIdxMode=One-based  errmode=Generate Error  FillMode=on  FillValues=0
  Variable Selector2 : dspindex/Variable Selector  NumInputs=2  rowsOrCols=Columns  IdxMode=Fixed  Elements=2  ZerOneIdxMode=One-based  errmode=Generate Error  FillMode=on  FillValues=0
  Variable Selector3 : dspindex/Variable Selector  NumInputs=2  rowsOrCols=Columns  IdxMode=Fixed  Elements=3  ZerOneIdxMode=One-based  errmode=Generate Error  FillMode=on  FillValues=0
  Variable Selector4 : dspindex/Variable Selector  NumInputs=2  rowsOrCols=Columns  IdxMode=Fixed  Elements=4  ZerOneIdxMode=One-based  errmode=Generate Error  FillMode=on  FillValues=0
  Variable Selector5 : dspindex/Variable Selector  NumInputs=2  rowsOrCols=Columns  IdxMode=Fixed  Elements=5  ZerOneIdxMode=One-based  errmode=Generate Error  FillMode=on  FillValues=0
  Variable Selector6 : dspindex/Variable Selector  NumInputs=2  rowsOrCols=Columns  IdxMode=Fixed  Elements=6  ZerOneIdxMode=One-based  errmode=Generate Error  FillMode=on  FillValues=0
  Variable Selector7 : dspindex/Variable Selector  NumInputs=1  rowsOrCols=Columns  IdxMode=Variable  Elements=1  ZerOneIdxMode=One-based  errmode=Generate Error  FillMode=on  FillValues=0
  eps_i : Outport
  wires:
  Variable Selector/1 -> Variable Selector3/1, Variable Selector4/1, Variable Selector6/1, Variable Selector5/1, Variable Selector2/1, Variable Selector1/1  "a(i)"
  x/1 -> Variable Selector7/1, Variable Selector2/2, Variable Selector3/2, Variable Selector4/2, Variable Selector6/2, Variable Selector5/2, Variable Selector1/2  "x"
  Constant/1 -> Variable Selector/1
  i/1 -> Variable Selector7/2, Variable Selector/3
  Variable Selector1/1 -> Divide/1  "a(i,j)"
  Variable Selector1/2 -> Subtract/1  "x(j)"
  Subtract/1 -> Divide/2
  Variable Selector2/2 -> Subtract1/1  "x(j)"
  Variable Selector2/1 -> Divide1/1  "a(i,j)"
  Subtract1/1 -> Divide1/2
  Variable Selector3/1 -> Divide2/1  "a(i,j)"
  Variable Selector3/2 -> Subtract2/1  "x(j)"
  Subtract2/1 -> Divide2/2
  Variable Selector4/1 -> Divide3/1  "a(i,j)"
  Variable Selector4/2 -> Subtract3/1  "x(j)"
  Subtract3/1 -> Divide3/2
  Variable Selector5/2 -> Subtract4/1  "x(j)"
  Subtract4/1 -> Divide4/2
  Variable Selector5/1 -> Divide4/1
  Variable Selector6/1 -> Divide5/1  "a(i,j)"
  Variable Selector7/1 -> Subtract6/2, Subtract5/2, Subtract4/2, Subtract3/2, Subtract2/2, Subtract1/2, Subtract/2  "x(i)"
  Variable Selector6/2 -> Subtract5/1  "x(j)"
  Subtract5/1 -> Divide5/2
  Divide2/1 -> Sum of Elements/3
  Divide1/1 -> Sum of Elements/2
  Divide5/1 -> Sum of Elements/6
  Divide4/1 -> Sum of Elements/5
  Divide3/1 -> Sum of Elements/4
  Divide/1 -> Sum of Elements/1
  Variable Selector/2 -> Divide6/1  "g(i)"
  Subtract6/1 -> Divide6/2
  x0/1 -> Subtract6/1
  Divide6/1 -> Sum/2
  Sum of Elements/1 -> Sum/1
  Sum/1 -> eps_i/1
  Constant1/1 -> Variable Selector/2

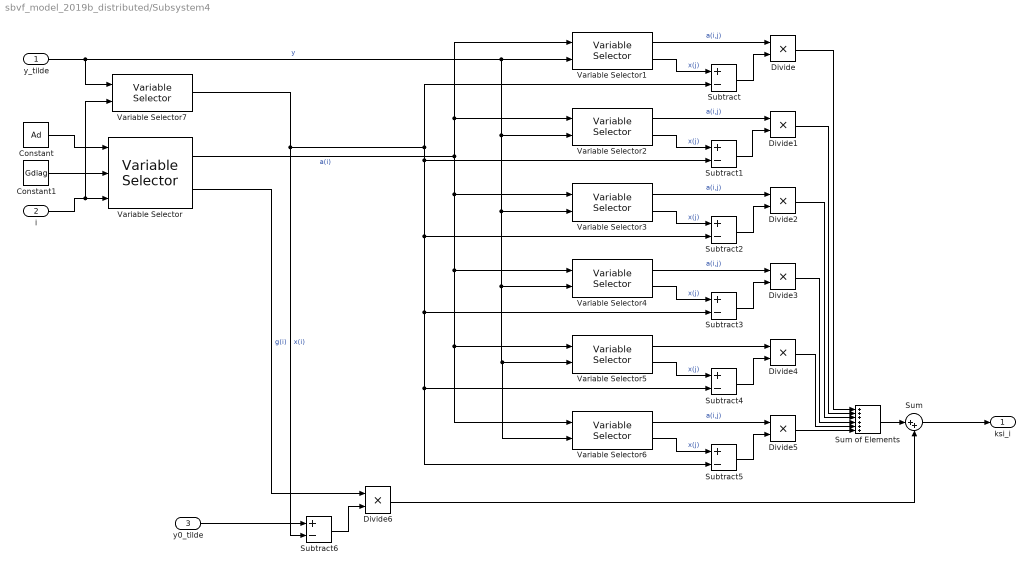
== system sbvf_model_2019b_distributed/Subsystem4 ==
  "y_tilde " : Inport
  i : Inport  Port=2
  "y0_tilde " : Inport  Port=3
  Constant : Constant  Value=Ad
  Constant1 : Constant  Value=Gdiag
  Divide{,1..6} (7 alike) : Product
  Subtract{,1..6} (7 alike) : Sum  Inputs=+-
  Sum : Sum  Inputs=|++
  Sum of Elements : Sum  Inputs=++++++
  Variable Selector : dspindex/Variable Selector  NumInputs=2  rowsOrCols=Rows  IdxMode=Variable  Elements=[1 3]  ZerOneIdxMode=One-based  errmode=Clip and Warn  FillMode=on  FillValues=0
  Variable Selector1 : dspindex/Variable Selector  NumInputs=2  rowsOrCols=Columns  IdxMode=Fixed  Elements=1  ZerOneIdxMode=One-based  errmode=Generate Error  FillMode=on  FillValues=0
  Variable Selector2 : dspindex/Variable Selector  NumInputs=2  rowsOrCols=Columns  IdxMode=Fixed  Elements=2  ZerOneIdxMode=One-based  errmode=Generate Error  FillMode=on  FillValues=0
  Variable Selector3 : dspindex/Variable Selector  NumInputs=2  rowsOrCols=Columns  IdxMode=Fixed  Elements=3  ZerOneIdxMode=One-based  errmode=Generate Error  FillMode=on  FillValues=0
  Variable Selector4 : dspindex/Variable Selector  NumInputs=2  rowsOrCols=Columns  IdxMode=Fixed  Elements=4  ZerOneIdxMode=One-based  errmode=Generate Error  FillMode=on  FillValues=0
  Variable Selector5 : dspindex/Variable Selector  NumInputs=2  rowsOrCols=Columns  IdxMode=Fixed  Elements=5  ZerOneIdxMode=One-based  errmode=Generate Error  FillMode=on  FillValues=0
  Variable Selector6 : dspindex/Variable Selector  NumInputs=2  rowsOrCols=Columns  IdxMode=Fixed  Elements=6  ZerOneIdxMode=One-based  errmode=Generate Error  FillMode=on  FillValues=0
  Variable Selector7 : dspindex/Variable Selector  NumInputs=1  rowsOrCols=Columns  IdxMode=Variable  Elements=1  ZerOneIdxMode=One-based  errmode=Generate Error  FillMode=on  FillValues=0
  ksi_i : Outport
  wires:
  Variable Selector/1 -> Variable Selector3/1, Variable Selector4/1, Variable Selector6/1, Variable Selector5/1, Variable Selector2/1, Variable Selector1/1  "a(i)"
  "y_tilde "/1 -> Variable Selector7/1, Variable Selector2/2, Variable Selector3/2, Variable Selector4/2, Variable Selector6/2, Variable Selector5/2, Variable Selector1/2  "y"
  Constant/1 -> Variable Selector/1
  i/1 -> Variable Selector7/2, Variable Selector/3
  Variable Selector1/1 -> Divide/1  "a(i,j)"
  Variable Selector1/2 -> Subtract/1  "x(j)"
  Subtract/1 -> Divide/2
  Variable Selector2/2 -> Subtract1/1  "x(j)"
  Variable Selector2/1 -> Divide1/1  "a(i,j)"
  Subtract1/1 -> Divide1/2
  Variable Selector3/1 -> Divide2/1  "a(i,j)"
  Variable Selector3/2 -> Subtract2/1  "x(j)"
  Subtract2/1 -> Divide2/2
  Variable Selector4/1 -> Divide3/1  "a(i,j)"
  Variable Selector4/2 -> Subtract3/1  "x(j)"
  Subtract3/1 -> Divide3/2
  Variable Selector5/2 -> Subtract4/1  "x(j)"
  Subtract4/1 -> Divide4/2
  Variable Selector5/1 -> Divide4/1
  Variable Selector6/1 -> Divide5/1  "a(i,j)"
  Variable Selector7/1 -> Subtract6/2, Subtract5/2, Subtract4/2, Subtract3/2, Subtract2/2, Subtract1/2, Subtract/2  "x(i)"
  Variable Selector6/2 -> Subtract5/1  "x(j)"
  Subtract5/1 -> Divide5/2
  Divide2/1 -> Sum of Elements/3
  Divide1/1 -> Sum of Elements/2
  Divide5/1 -> Sum of Elements/6
  Divide4/1 -> Sum of Elements/5
  Divide3/1 -> Sum of Elements/4
  Divide/1 -> Sum of Elements/1
  Variable Selector/2 -> Divide6/1  "g(i)"
  Subtract6/1 -> Divide6/2
  "y0_tilde "/1 -> Subtract6/1
  Divide6/1 -> Sum/2
  Sum of Elements/1 -> Sum/1
  Sum/1 -> ksi_i/1
  Constant1/1 -> Variable Selector/2

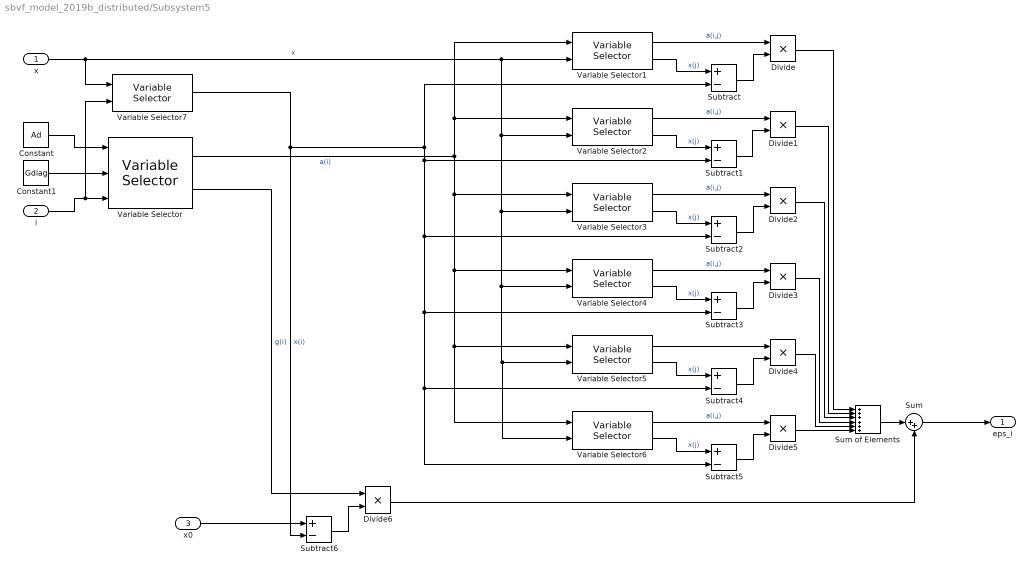
== system sbvf_model_2019b_distributed/Subsystem5 ==
  x : Inport
  i : Inport  Port=2
  x0 : Inport  Port=3
  Constant : Constant  Value=Ad
  Constant1 : Constant  Value=Gdiag
  Divide{,1..6} (7 alike) : Product
  Subtract{,1..6} (7 alike) : Sum  Inputs=+-
  Sum : Sum  Inputs=|++
  Sum of Elements : Sum  Inputs=++++++
  Variable Selector : dspindex/Variable Selector  NumInputs=2  rowsOrCols=Rows  IdxMode=Variable  Elements=[1 3]  ZerOneIdxMode=One-based  errmode=Clip and Warn  FillMode=on  FillValues=0
  Variable Selector1 : dspindex/Variable Selector  NumInputs=2  rowsOrCols=Columns  IdxMode=Fixed  Elements=1  ZerOneIdxMode=One-based  errmode=Generate Error  FillMode=on  FillValues=0
  Variable Selector2 : dspindex/Variable Selector  NumInputs=2  rowsOrCols=Columns  IdxMode=Fixed  Elements=2  ZerOneIdxMode=One-based  errmode=Generate Error  FillMode=on  FillValues=0
  Variable Selector3 : dspindex/Variable Selector  NumInputs=2  rowsOrCols=Columns  IdxMode=Fixed  Elements=3  ZerOneIdxMode=One-based  errmode=Generate Error  FillMode=on  FillValues=0
  Variable Selector4 : dspindex/Variable Selector  NumInputs=2  rowsOrCols=Columns  IdxMode=Fixed  Elements=4  ZerOneIdxMode=One-based  errmode=Generate Error  FillMode=on  FillValues=0
  Variable Selector5 : dspindex/Variable Selector  NumInputs=2  rowsOrCols=Columns  IdxMode=Fixed  Elements=5  ZerOneIdxMode=One-based  errmode=Generate Error  FillMode=on  FillValues=0
  Variable Selector6 : dspindex/Variable Selector  NumInputs=2  rowsOrCols=Columns  IdxMode=Fixed  Elements=6  ZerOneIdxMode=One-based  errmode=Generate Error  FillMode=on  FillValues=0
  Variable Selector7 : dspindex/Variable Selector  NumInputs=1  rowsOrCols=Columns  IdxMode=Variable  Elements=1  ZerOneIdxMode=One-based  errmode=Generate Error  FillMode=on  FillValues=0
  eps_i : Outport
  wires:
  Variable Selector/1 -> Variable Selector3/1, Variable Selector4/1, Variable Selector6/1, Variable Selector5/1, Variable Selector2/1, Variable Selector1/1  "a(i)"
  x/1 -> Variable Selector7/1, Variable Selector2/2, Variable Selector3/2, Variable Selector4/2, Variable Selector6/2, Variable Selector5/2, Variable Selector1/2  "x"
  Constant/1 -> Variable Selector/1
  i/1 -> Variable Selector7/2, Variable Selector/3
  Variable Selector1/1 -> Divide/1  "a(i,j)"
  Variable Selector1/2 -> Subtract/1  "x(j)"
  Subtract/1 -> Divide/2
  Variable Selector2/2 -> Subtract1/1  "x(j)"
  Variable Selector2/1 -> Divide1/1  "a(i,j)"
  Subtract1/1 -> Divide1/2
  Variable Selector3/1 -> Divide2/1  "a(i,j)"
  Variable Selector3/2 -> Subtract2/1  "x(j)"
  Subtract2/1 -> Divide2/2
  Variable Selector4/1 -> Divide3/1  "a(i,j)"
  Variable Selector4/2 -> Subtract3/1  "x(j)"
  Subtract3/1 -> Divide3/2
  Variable Selector5/2 -> Subtract4/1  "x(j)"
  Subtract4/1 -> Divide4/2
  Variable Selector5/1 -> Divide4/1
  Variable Selector6/1 -> Divide5/1  "a(i,j)"
  Variable Selector7/1 -> Subtract6/2, Subtract5/2, Subtract4/2, Subtract3/2, Subtract2/2, Subtract1/2, Subtract/2  "x(i)"
  Variable Selector6/2 -> Subtract5/1  "x(j)"
  Subtract5/1 -> Divide5/2
  Divide2/1 -> Sum of Elements/3
  Divide1/1 -> Sum of Elements/2
  Divide5/1 -> Sum of Elements/6
  Divide4/1 -> Sum of Elements/5
  Divide3/1 -> Sum of Elements/4
  Divide/1 -> Sum of Elements/1
  Variable Selector/2 -> Divide6/1  "g(i)"
  Subtract6/1 -> Divide6/2
  x0/1 -> Subtract6/1
  Divide6/1 -> Sum/2
  Sum of Elements/1 -> Sum/1
  Sum/1 -> eps_i/1
  Constant1/1 -> Variable Selector/2

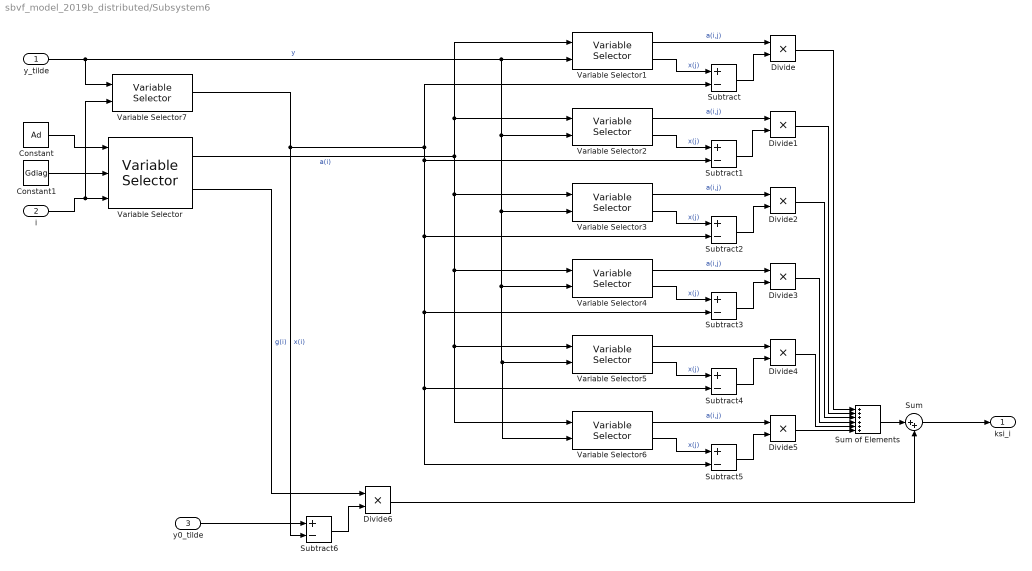
== system sbvf_model_2019b_distributed/Subsystem6 ==
  "y_tilde " : Inport
  i : Inport  Port=2
  "y0_tilde " : Inport  Port=3
  Constant : Constant  Value=Ad
  Constant1 : Constant  Value=Gdiag
  Divide{,1..6} (7 alike) : Product
  Subtract{,1..6} (7 alike) : Sum  Inputs=+-
  Sum : Sum  Inputs=|++
  Sum of Elements : Sum  Inputs=++++++
  Variable Selector : dspindex/Variable Selector  NumInputs=2  rowsOrCols=Rows  IdxMode=Variable  Elements=[1 3]  ZerOneIdxMode=One-based  errmode=Clip and Warn  FillMode=on  FillValues=0
  Variable Selector1 : dspindex/Variable Selector  NumInputs=2  rowsOrCols=Columns  IdxMode=Fixed  Elements=1  ZerOneIdxMode=One-based  errmode=Generate Error  FillMode=on  FillValues=0
  Variable Selector2 : dspindex/Variable Selector  NumInputs=2  rowsOrCols=Columns  IdxMode=Fixed  Elements=2  ZerOneIdxMode=One-based  errmode=Generate Error  FillMode=on  FillValues=0
  Variable Selector3 : dspindex/Variable Selector  NumInputs=2  rowsOrCols=Columns  IdxMode=Fixed  Elements=3  ZerOneIdxMode=One-based  errmode=Generate Error  FillMode=on  FillValues=0
  Variable Selector4 : dspindex/Variable Selector  NumInputs=2  rowsOrCols=Columns  IdxMode=Fixed  Elements=4  ZerOneIdxMode=One-based  errmode=Generate Error  FillMode=on  FillValues=0
  Variable Selector5 : dspindex/Variable Selector  NumInputs=2  rowsOrCols=Columns  IdxMode=Fixed  Elements=5  ZerOneIdxMode=One-based  errmode=Generate Error  FillMode=on  FillValues=0
  Variable Selector6 : dspindex/Variable Selector  NumInputs=2  rowsOrCols=Columns  IdxMode=Fixed  Elements=6  ZerOneIdxMode=One-based  errmode=Generate Error  FillMode=on  FillValues=0
  Variable Selector7 : dspindex/Variable Selector  NumInputs=1  rowsOrCols=Columns  IdxMode=Variable  Elements=1  ZerOneIdxMode=One-based  errmode=Generate Error  FillMode=on  FillValues=0
  ksi_i : Outport
  wires:
  Variable Selector/1 -> Variable Selector3/1, Variable Selector4/1, Variable Selector6/1, Variable Selector5/1, Variable Selector2/1, Variable Selector1/1  "a(i)"
  "y_tilde "/1 -> Variable Selector7/1, Variable Selector2/2, Variable Selector3/2, Variable Selector4/2, Variable Selector6/2, Variable Selector5/2, Variable Selector1/2  "y"
  Constant/1 -> Variable Selector/1
  i/1 -> Variable Selector7/2, Variable Selector/3
  Variable Selector1/1 -> Divide/1  "a(i,j)"
  Variable Selector1/2 -> Subtract/1  "x(j)"
  Subtract/1 -> Divide/2
  Variable Selector2/2 -> Subtract1/1  "x(j)"
  Variable Selector2/1 -> Divide1/1  "a(i,j)"
  Subtract1/1 -> Divide1/2
  Variable Selector3/1 -> Divide2/1  "a(i,j)"
  Variable Selector3/2 -> Subtract2/1  "x(j)"
  Subtract2/1 -> Divide2/2
  Variable Selector4/1 -> Divide3/1  "a(i,j)"
  Variable Selector4/2 -> Subtract3/1  "x(j)"
  Subtract3/1 -> Divide3/2
  Variable Selector5/2 -> Subtract4/1  "x(j)"
  Subtract4/1 -> Divide4/2
  Variable Selector5/1 -> Divide4/1
  Variable Selector6/1 -> Divide5/1  "a(i,j)"
  Variable Selector7/1 -> Subtract6/2, Subtract5/2, Subtract4/2, Subtract3/2, Subtract2/2, Subtract1/2, Subtract/2  "x(i)"
  Variable Selector6/2 -> Subtract5/1  "x(j)"
  Subtract5/1 -> Divide5/2
  Divide2/1 -> Sum of Elements/3
  Divide1/1 -> Sum of Elements/2
  Divide5/1 -> Sum of Elements/6
  Divide4/1 -> Sum of Elements/5
  Divide3/1 -> Sum of Elements/4
  Divide/1 -> Sum of Elements/1
  Variable Selector/2 -> Divide6/1  "g(i)"
  Subtract6/1 -> Divide6/2
  "y0_tilde "/1 -> Subtract6/1
  Divide6/1 -> Sum/2
  Sum of Elements/1 -> Sum/1
  Sum/1 -> ksi_i/1
  Constant1/1 -> Variable Selector/2
